simulink model "TSat3_Send_Receive_Data"  (Simulink 6.6)
settings: Solver=FixedStepDiscrete  SolverMode=SingleTasking  StartTime=0.0  StopTime=10000  FixedStep=.1  RelTol=1e-3
StopFcn:
  | PlotSimout
settings Model: Creator=rob  LastModifiedBy=Administrator  ExtModeAutoUpdateStatusClock=off
settings DataIOCC: SignalLoggingName=sigsOut
settings OptimizationCC: InlineInvariantSignals=on
settings DebuggingCC: SignalResolutionControl=TryResolveAllWithWarning  SolverPrmCheckMsg=none  MultiTaskDSMMsg=warning  MultiTaskCondExecSysMsg=none  StrictBusMsg=None
settings HardwareCC: TargetUnknown=on
settings RTWCC: IncludeERTFirstTime=on

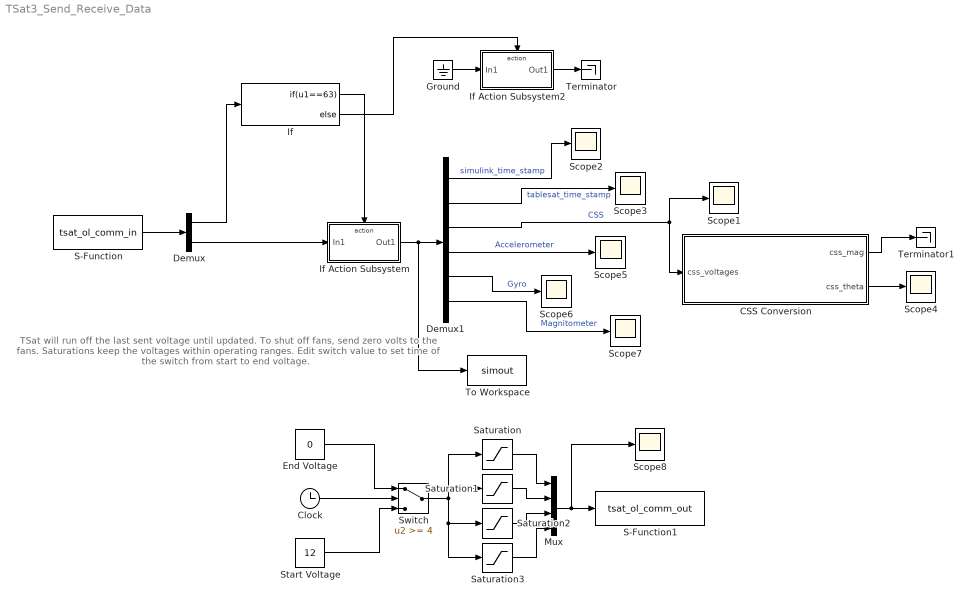
== system TSat3_Send_Receive_Data ==
  note: TSat will run off the last sent voltage until updated.
      | To shut off fans, send zero volts to the fans.
      |
      | Saturations keep the voltages within operating ranges.
      |
      | Edit switch value to set time of the switch from start to end voltage.
  CSS Conversion : Stateflow chart
  Clock : Clock
      settings: Decimation=10
  Demux : Demux  Outputs=[1;-1]
  Demux1 : Demux  Outputs=[1;1;6;4;1;3]
  End Voltage : Constant  Value=0
  Ground : Ground
  If : If  IfExpression=u1==63
  If Action Subsystem : Subsystem  TreatAsAtomicUnit=on
  If Action Subsystem2 : Subsystem  TreatAsAtomicUnit=on
  Mux : Mux
  S-Function : S-Function  FunctionName=tsat_ol_comm_in
  S-Function1 : S-Function  FunctionName=tsat_ol_comm_out
  Saturation : Saturate  UpperLimit=0  LowerLimit=0
  Saturation1 : Saturate  UpperLimit=12  LowerLimit=0
  Saturation2 : Saturate  UpperLimit=0  LowerLimit=0
  Saturation3 : Saturate  UpperLimit=0  LowerLimit=0
  Scope{1..8} (8 alike) : Scope
      Scope1 settings: TimeRange=10000  YMin=0.15  YMax=0.6  SaveName=ScopeData3
      Scope2 settings: TimeRange=10  YMin=0.7  YMax=2
      Scope3 settings: YMin=990.5  YMax=991.7  SaveName=ScopeData2
      Scope4 settings: TimeRange=8  YMin=0  YMax=7  SaveName=ScopeData7
      Scope5 settings: TimeRange=18  YMin=2.4  YMax=2.65  SaveName=ScopeData4
      Scope6 settings: SaveName=ScopeData5
      Scope7 settings: TimeRange=9  YMin=2  YMax=2.7  SaveName=ScopeData6
      Scope8 settings: YMin=-1  YMax=1
  Start Voltage : Constant  Value=12
  Switch : Switch  Threshold=4
  Terminator : Terminator
  Terminator1 : Terminator
  To Workspace : ToWorkspace  VariableName=simout  SampleTime=-1  SaveFormat=Array
  wires:
  If/1 -> If Action Subsystem/Action
  If/2 -> If Action Subsystem2/Action
  Demux/1 -> If/1
  S-Function/1 -> Demux/1
  If Action Subsystem2/1(Out1) -> Terminator/1
  Demux/2 -> If Action Subsystem/1(In1)
  Ground/1 -> If Action Subsystem2/1(In1)
  If Action Subsystem/1(Out1) -> Demux1/1, To Workspace/1
  Demux1/1 -> Scope2/1  "simulink_time_stamp"
  Demux1/2 -> Scope3/1  "tablesat_time_stamp"
  Demux1/3 -> CSS Conversion/1(css_voltages), Scope1/1  "CSS"
  Demux1/4 -> Scope5/1  "Accelerometer"
  Demux1/5 -> Scope6/1  "Gyro"
  Demux1/6 -> Scope7/1  "Magnitometer"
  Saturation/1 -> Mux/1
  Saturation1/1 -> Mux/2
  Saturation2/1 -> Mux/3
  Saturation3/1 -> Mux/4
  Mux/1 -> S-Function1/1, Scope8/1
  End Voltage/1 -> Switch/1
  Start Voltage/1 -> Switch/3
  Clock/1 -> Switch/2
  Switch/1 -> Saturation/1, Saturation1/1, Saturation2/1, Saturation3/1
  CSS Conversion/1(css_mag) -> Terminator1/1
  CSS Conversion/2(css_theta) -> Scope4/1

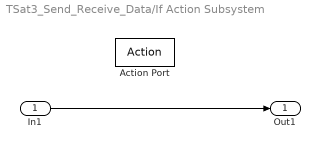
== system TSat3_Send_Receive_Data/If Action Subsystem ==
  In1 : Inport
  Action Port : ActionPort  ActionType=then
  Out1 : Outport
  wires:
  In1/1 -> Out1/1

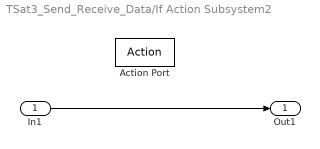
== system TSat3_Send_Receive_Data/If Action Subsystem2 ==
  In1 : Inport
  Action Port : ActionPort  ActionType=else
  Out1 : Outport
  wires:
  In1/1 -> Out1/1

== matlab function CSS Conversion ==
  data: css_voltages input inherited; css_mag output inherited; css_theta output inherited
function [ css_mag, css_theta ] = css_to_theta( css_voltages )
%CSS_TO_THETA uses the six sun sensors to find the direction to the largest
%source of light.
%   Inputs:  vector of 6 css voltages.  CSS 1 is assumed to be zero
%   degrees.  An offset may be added to this code if a different zero is
%   needed.
%   
%   Outputs:  Using a resultant force style analysis.  The resultant
%   magnitude showing the strength of the signal and the resultant angle
%   theta are returned.
%
css_x=0;
css_y=0;
for n = 1:size(css_voltages,1)
    css_x = css_x + cos((n-1)*pi()/3)*css_voltages(n);
    css_y = css_y + sin((n-1)*pi()/3)*css_voltages(n);
end
css_mag = (css_x^2+css_y^2)^0.5;
css_theta = atan(css_y/css_x);
if css_x < 0
    css_theta = css_theta+pi();
end
if css_theta < 0
    css_theta = css_theta + 2*pi();
end
